simulink model "test2"  (R2019b)
settings: Solver=VariableStepAuto  StartTime=0.0  StopTime=10.0  RelTol=1e-3
values from neighbouring files (symbols this model uses):
  x = [200,1,20,0,0]    [SBW_main.m]    (also in Single_Obj_pso.m = abs(x) .*[1000, 10, 100,1,1]; multi_obj_mopso.m = abs(x) .*[1000, 10, 100,1,1]; single_obj_fminsearch.m = OrderedList(); single_obj_nelder_and_mead.m = zeros(nrParam,nrParam+1))
settings Model: Creator=Tan Eng Meng  LastModifiedBy=Tan Eng Meng

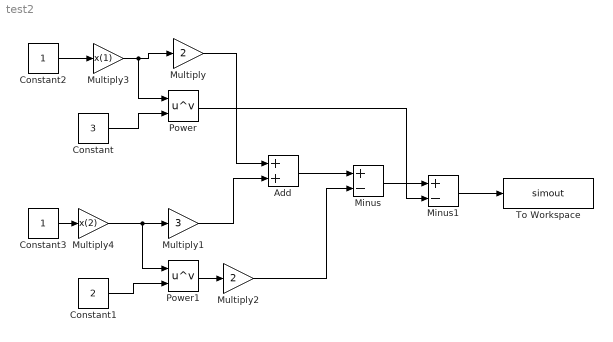
== system test2 ==
  Add : Sum
  Constant : Constant  Value=3
  Constant1 : Constant  Value=2
  Constant2 : Constant
  Constant3 : Constant
  Minus : Sum  Inputs=+-
  Minus1 : Sum  Inputs=+-
  Multiply : Gain  Gain=2
  Multiply1 : Gain  Gain=3
  Multiply2 : Gain  Gain=2
  Multiply3 : Gain  Gain=x(1)
  Multiply4 : Gain  Gain=x(2)
  Power : Math  Operator=pow  SignedPower=off  SaturateOnIntegerOverflow=on
  Power1 : Math  Operator=pow  SignedPower=off  SaturateOnIntegerOverflow=on
  To Workspace : ToWorkspace  VariableName=simout  SaveFormat=Timeseries  SampleTime=-1
  wires:
  Constant/1 -> Power/2
  Multiply4/1 -> Power1/1, Multiply1/1
  Constant1/1 -> Power1/2
  Power1/1 -> Multiply2/1
  Multiply/1 -> Add/1
  Multiply1/1 -> Add/2
  Add/1 -> Minus/1
  Multiply2/1 -> Minus/2
  Minus/1 -> Minus1/1
  Power/1 -> Minus1/2
  Minus1/1 -> To Workspace/1
  Constant2/1 -> Multiply3/1
  Multiply3/1 -> Power/1, Multiply/1
  Constant3/1 -> Multiply4/1
